simulink model "Steuerung"  (R2018a)
settings: Solver=ode1  StartTime=0.0  StopTime=inf  FixedStep=1/10  RelTol=1e-3  EnableMultiTasking=on
undefined symbols (not defined in the file or in its folder): gray
libraries: simulink x3, visiontransforms x2, PiCar_library x1, visiontextngfix x1, visionanalysis x1, visionstatistics x1, embdlinuxlib x1, visionsinks x1
settings Model: SimulationMode=external  Creator=raspberry  LastModifiedBy=jonaseckhoff
settings SolverCC: PositivePriorityOrder=on
settings OptimizationCC: PassReuseOutputArgsAs=Individual arguments  MaxStackSize=64
settings DebuggingCC: ParameterTunabilityLossMsg=error
settings HardwareCC: ProdBitPerPointer=32  ProdBitPerSizeT=32  ProdBitPerPtrDiffT=32  ProdLargestAtomicInteger=Long  ProdLargestAtomicFloat=Double  ProdWordSize=32  ProdHWDeviceType=ARM Compatible->ARM Cortex
settings SFSimCC: MATLABDynamicMemAlloc=off
settings RTWCC: SystemTargetFile=ert.tlc  HardwareBoard=Raspberry Pi  TLCOptions="-aInlineSetEventsForThisBaseRateFcn=TLC_FALSE -aSuppressMultiTaskScheduler=TLC_FALSE  -aRateBasedStepFcn=0"  TemplateMakefile=ert_default_tmf  Toolchain=GNU GCC Raspberry Pi
settings RTWCC: CustomTerminator=|
  | /* Send ALL_LED_OFF Signal to all PWM driver chip address
  | See PCA9685 user manual, section 7.3.4
  | Set Chip in sleep mode, section 7.3.1
  | Reset the PWM ON/OFF states for all LEDs */
  | 
  | int fd;
  | 
  | fd = wiringPiI2CSetup(0x70);
  | wiringPiI2CWriteReg8(fd, 0x00, 0x11); // sleep mode
  | wiringPiI2CWriteReg8(fd, 0xFD, 0x10); // all LED off
  | wiringPiI2CWriteReg8(fd, 0xFC, 0x00);
  | wiringPiI2CWriteReg8(fd, 0xFB, 0x00);
  | wiringPiI2CWriteReg8(fd, 0xFA, 0x00);
settings CodeAppCC: ForceParamTrailComments=on  IgnoreCustomStorageClasses=off  OperatorAnnotations=on  SimulinkDataObjDesc=on  SFDataObjDesc=on  MATLABFcnDesc=on  InsertBlockDesc=on  StateflowObjectComments=on  MATLABSourceComments=on
settings ERTTargetCC: SupportVariableSizeSignals=on

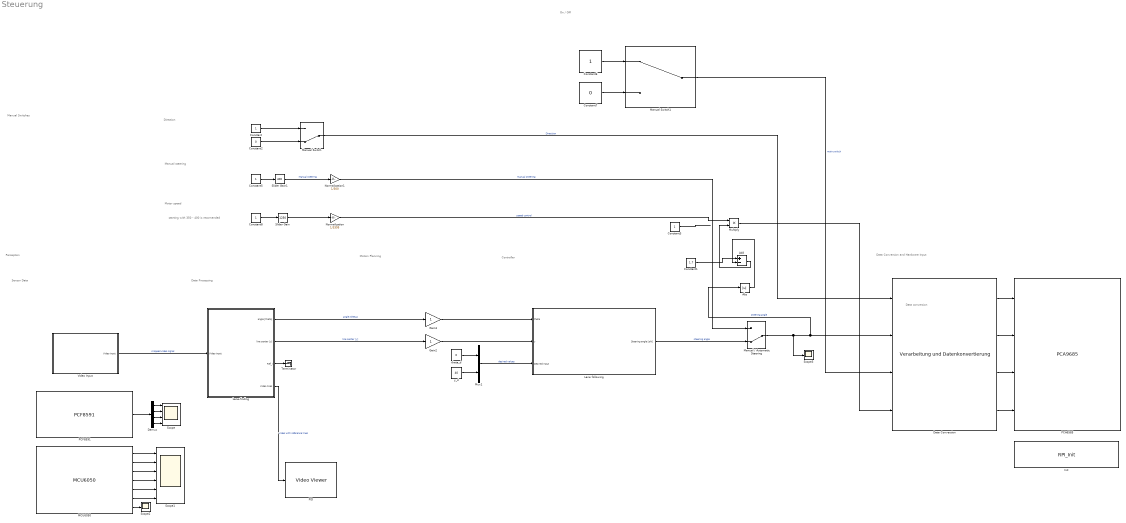
== system Steuerung ==
  note: starting with 350 - 400 is recomended
  note: Data Conversion and Hardware Input
  note: Data conversion
  note: Manual Switches
  note: Motion Planning
  note: Perception
  note: Controller
  note: Data Processing
  note: Sensor Data
  note: Manual steering
  note: Motor speed
  note: Direction
  note: On / Off
  Abs : Abs
  Add : Sum  Inputs=+-
  Constant{,3,5..6,8} (5 alike) : Constant
  Constant1 : Constant  Value=1.7
  Constant2 : Constant  Value=0
  Constant7 : Constant  Value=0
  Data Conversion : PiCar_library/Verarbeitung und Datenkonvertierung
      link override Gain1: Gain=340
  Demux : Demux
  Gain2 : Gain
  Gain3 : Gain
  Init : S-Function  Priority=1  InitFcn=try, set_param(gcb,'FunctionName','RPI_Init'), end  FunctionName=RPI_Init  SFunctionModules=RPI_Init_wrapper  SFunctionDeploymentMode=off  EnableBusSupport=off  mask(S-Function Builder){}
      mask help: Simulink:masks:SFunctionBuilder_MD
      mask init:
      | val = [[.9  0.75 0.75 1 1 .9 .9 1]',[1 1 0.75 0.75 .9 .9 1 .9]'];try , sys = get_param(gcb,'SfunBuilderFcnName');if isempty(sys), sys = get_param(gcb,'FunctionName'); end,catch, sys = get_param(gcb,'FunctionName'); end
      settings: CopyFcn=set_param(gcbh,'LinkStatus','none')  PreSaveFcn=try, set_param(gcb,'FunctionName','RPI_Init'), end  OpenFcn=sfunctionwizard(gcbh)
      mask Display:
      | plot(val(:,1),val(:,2))
      | disp(sys)
  Lane following : Subsystem  AncestorBlock=PiCar_library/Lane following
  Lane-finding : Subsystem  AncestorBlock=PiCar_library/Lane-finding
  MCU6050 : S-Function  InitFcn=try, set_param(gcb,'FunctionName','MCU6050'), end  FunctionName=MCU6050  SFunctionModules=MCU6050_wrapper  SFunctionDeploymentMode=off  EnableBusSupport=off  mask(S-Function Builder){}
      mask help: Simulink:masks:SFunctionBuilder_MD
      mask init: same as Steuerung/Init
      settings: CopyFcn=set_param(gcbh,'LinkStatus','none')  PreSaveFcn=try, set_param(gcb,'FunctionName','MCU6050'), end  OpenFcn=sfunctionwizard(gcbh)
      mask Display: plot(val(:,1),val(:,2)),disp(sys), port_label('output',1,'ax'), port_label('output',2,'ay'), port_label('output',3,'az'), port_label('output',4,'omx'), port_label('output',5,'omy'), port_label('output',6,'omz'), port_label('output',7,'temp')
  Manual / Automatic Steering : ManualSwitch  CurrentSetting=0
  Manual Switch : ManualSwitch  CurrentSetting=0
  Manual Switch1 : ManualSwitch
  Multiply : Product
  Mux1 : Mux  Inputs=2
  Normalization : Gain  Gain=1/3395
  Normalization1 : Gain  Gain=1/300
  PCA6585 : S-Function  InitFcn=try, set_param(gcb,'FunctionName','PCA9685'), end  FunctionName=PCA9685  SFunctionModules=PCA9685_wrapper  SFunctionDeploymentMode=off  EnableBusSupport=off  mask(S-Function Builder){}
      mask help: Simulink:masks:SFunctionBuilder_MD
      mask init: same as Steuerung/Init
      settings: CopyFcn=set_param(gcbh,'LinkStatus','none')  PreSaveFcn=try, set_param(gcb,'FunctionName','PCA9685'), end  OpenFcn=sfunctionwizard(gcbh)
      mask Display: plot(val(:,1),val(:,2)),disp(sys), port_label('input',1,'IN_1'), port_label('input',2,'IN_2'), port_label('input',3,'PWM'), port_label('input',4,'SERVO')
  PCF8591 : S-Function  InitFcn=try, set_param(gcb,'FunctionName','PCF8591'), end  FunctionName=PCF8591  SFunctionModules=PCF8591_wrapper  SFunctionDeploymentMode=off  EnableBusSupport=off  mask(S-Function Builder){}
      mask help: Simulink:masks:SFunctionBuilder_MD
      mask init: same as Steuerung/Init
      settings: CopyFcn=set_param(gcbh,'LinkStatus','none')  PreSaveFcn=try, set_param(gcb,'FunctionName','PCF8591'), end  OpenFcn=sfunctionwizard(gcbh)
      mask Display: plot(val(:,1),val(:,2)),disp(sys), port_label('output',1,'PCF8591_out')
  PID : VideoViewer  colormapValue=gray(256)  FigPos=[241 558 555 306]
  Scope : Scope  NumInputPorts=4
  Scope1 : Scope  NumInputPorts=6
  Scope2 : Scope
  Scope3 : Scope
  Slider Gain : simulink/Math Operations/Slider Gain  gain=1250  low=0  high=3395
  Slider Gain1 : simulink/Math Operations/Slider Gain  gain=400  low=-400  high=400
  Terminator : Terminator
  Video Input : Subsystem  AncestorBlock=PiCar_library/Video Input
  theta_d : Constant  Value=0
  y_d : Constant  Value=40
  wires:
  Constant/1 -> Manual Switch/1
  Constant2/1 -> Manual Switch/2
  Constant7/1 -> Manual Switch1/2
  Constant6/1 -> Manual Switch1/1
  Constant8/1 -> Slider Gain/1
  Slider Gain1/1 -> Normalization1/1  "Manual steering"
  Constant5/1 -> Slider Gain1/1
  Lane-finding/2(line center [y]) -> Gain2/1  "line center [y]"
  Demux/3 -> Scope/3
  Demux/4 -> Scope/4
  PCF8591/1 -> Demux/1
  MCU6050/2 -> Scope1/2
  MCU6050/3 -> Scope1/3
  MCU6050/1 -> Scope1/1
  MCU6050/4 -> Scope1/4
  MCU6050/5 -> Scope1/5
  MCU6050/6 -> Scope1/6
  MCU6050/7 -> Scope2/1
  Manual Switch/1 -> Data Conversion/1  "Direction"
  Manual / Automatic Steering/1 -> Abs/1, Data Conversion/2, Scope3/1  "steering angle"
  Manual Switch1/1 -> Data Conversion/3  "main switch"
  Data Conversion/1 -> PCA6585/1
  Data Conversion/2 -> PCA6585/2
  Data Conversion/3 -> PCA6585/3
  Data Conversion/4 -> PCA6585/4
  Lane-finding/1(angle [theta]) -> Gain3/1  "angle [theta]"
  Slider Gain/1 -> Normalization/1
  Lane-finding/3(Ref_I) -> Terminator/1
  Lane-finding/4(Video lines) -> PID/1  "video with reference lines"
  Normalization/1 -> Multiply/1  "speed control"
  y_d/1 -> Mux1/2
  theta_d/1 -> Mux1/1
  Mux1/1 -> Lane following/3(Desired input)  "desired values"
  Normalization1/1 -> Manual / Automatic Steering/1  "manual steering"
  Demux/1 -> Scope/1
  Demux/2 -> Scope/2
  Gain3/1 -> Lane following/1(theta)
  Gain2/1 -> Lane following/2(y)
  Lane following/1(Steering angle [phi]) -> Manual / Automatic Steering/2  "steering angle"
  Video Input/1(Video Input) -> Lane-finding/1(Video input)  "cropped video signal"
  Abs/1 -> Add/2
  Constant1/1 -> Add/1
  Multiply/1 -> Data Conversion/4
  Constant3/1 -> ?
  Add/1 -> Multiply/2

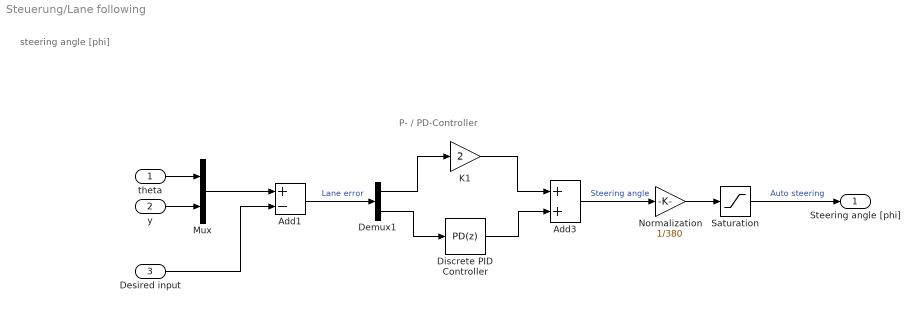
== system Steuerung/Lane following ==
  note: steering angle [phi]
  note: P- / PD-Controller
  theta : Inport
  y : Inport  Port=2
  Desired input : Inport  Port=3
  Add1 : Sum  Inputs=+-
  Add3 : Sum
  Demux1 : Demux  Outputs=2
  Discrete PID Controller : simulink/Continuous/PID Controller  Controller=PD  TimeDomain=Discrete-time  SampleTime=-1  IntegratorMethod=Forward Euler  FilterMethod=Forward Euler  Form=Parallel  UseFilter=off  ControllerParametersSource=internal  P=18  I=1.5  D=1.5  N=100  InitialConditionSource=internal  InitialConditionForIntegrator=0  InitialConditionForFilter=0  ExternalReset=none  LimitOutput=off  UpperSaturationLimit=inf  LowerSaturationLimit=-inf  LinearizeAsGain=off  AntiWindupMode=none  Kb=1  TrackingMode=off  Kt=1  PParamMin=[]  PParamMax=[]  IParamMin=[]  IParamMax=[]  DParamMin=[]  DParamMax=[]  NParamMin=[]  NParamMax=[]  KbParamMin=[]  KbParamMax=[]  KtParamMin=[]  KtParamMax=[]  POutMin=[]  POutMax=[]  IOutMin=[]  IOutMax=[]  DOutMin=[]  DOutMax=[]  NOutMin=[]  NOutMax=[]  KbOutMin=[]  KbOutMax=[]  KtOutMin=[]  KtOutMax=[]  IntegratorOutMin=[]  IntegratorOutMax=[]  FilterOutMin=[]  FilterOutMax=[]  SumOutMin=[]  SumOutMax=[]  SumI1OutMin=[]  SumI1OutMax=[]  SumI2OutMin=[]  SumI2OutMax=[]  SumI3OutMin=[]  SumI3OutMax=[]  SumDOutMin=[]  SumDOutMax=[]  SaturationOutMin=[]  SaturationOutMax=[]  IntegratorContinuousStateAttributes=''  IntegratorStateMustResolveToSignalObject=off  IntegratorRTWStateStorageClass=Auto  FilterContinuousStateAttributes=''  FilterStateMustResolveToSignalObject=off  FilterRTWStateStorageClass=Auto  DifferentiatorICPrevScaledInput=0  DifferentiatorOutMin=[]  DifferentiatorOutMax=[]  FilterDiffOutCoefMin=[]  FilterDiffOutCoefMax=[]  SumDenOutMin=[]  SumDenOutMax=[]  SumNumOutMin=[]  SumNumOutMax=[]  ReciprocalOutMin=[]  ReciprocalOutMax=[]  DivideOutMin=[]  DivideOutMax=[]  TunerSelectOption=Transfer Function Based (PID Tuner App)
  K1 : Gain  Gain=2
  Mux : Mux  Inputs=2
  Normalization : Gain  Gain=1/380
  Saturation : Saturate  UpperLimit=1  LowerLimit=-1
  Steering angle [phi] : Outport
  wires:
  theta/1 -> Mux/1
  y/1 -> Mux/2
  Mux/1 -> Add1/1
  Desired input/1 -> Add1/2
  Saturation/1 -> Steering angle [phi]/1  "Auto steering"
  Add3/1 -> Normalization/1  "Steering angle"
  Discrete PID Controller/1 -> Add3/2
  Demux1/2 -> Discrete PID Controller/1
  Add1/1 -> Demux1/1  "Lane error"
  Demux1/1 -> K1/1
  K1/1 -> Add3/1
  Normalization/1 -> Saturation/1

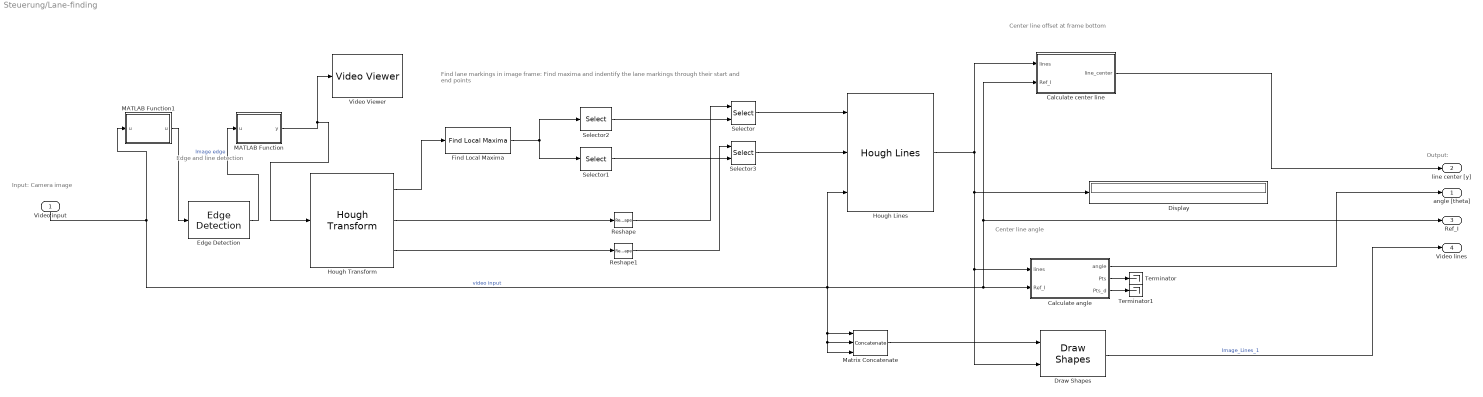
== system Steuerung/Lane-finding ==
  note: Output:
  note: Input: Camera image
  note: Edge and line detection
  note: Find lane markings in image frame:
      | Find maxima and indentify the lane markings through their start and end points
  note: Center line angle
  note: Center line offset at frame bottom
  Video input : Inport
  Calculate angle : MATLAB Function  TreatAsAtomicUnit=on
  Calculate center line : MATLAB Function  TreatAsAtomicUnit=on
  Display : Display
  Draw Shapes : visiontextngfix/Draw Shapes  shape=Lines  fill=off  lineWidth=1  fillClrSource=Specify via dialog  display=User-specified value  intensity=200  color=[0 0 255]  opacity=0.6  viewport=Entire image  antialiasing=off  inType=Obsolete  imagePorts=One multidimensional signal  prodOutputMode=Binary point scaling  prodOutputWordLength=32  prodOutputFracLength=14  memoryMode=Specify word length  memoryWordLength=16  memoryFracLength=14  roundingMode=Floor  overflowMode=off
      settings: SourceProductName=Computer Vision System Toolbox
  Edge Detection : visionanalysis/Edge Detection  method=Sobel  outputType=Binary image  userDefinedThreshold=off  thresholdSource=Input port  threshold=20  thresholdTuning=4  edgeThinning=off  threshold_canny=[0.25 0.60]  autoPercent=70  sigma=1  roundingMode=Floor  overflowMode=off  prodOutputMode=Binary point scaling  prodOutputWordLength=32  prodOutputFracLength=8  prodOutputSlope=2^-8  accumSlope=2^-8  outputSlope=2^-4
      settings: SourceProductName=Computer Vision System Toolbox  SourceProductBaseCode=VP
  Find Local Maxima : visionstatistics/Find Local Maxima  num_peaks=2  nhood_size=[5 7]  src_thresh=Obsolete9b  src_thresh_inuse=Specify via dialog  threshold=10  inputIsHough=off  dt_peak=uint32  isOutVarDim=on  dt_count=uint32
      settings: SourceProductName=Computer Vision System Toolbox  SourceProductBaseCode=VP
  Hough Lines : visiontransforms/Hough Lines  sineCompMethod=Trigonometric function  thetaRes=pi/180  firstCoeffMode=Specify word length  firstCoeffWordLength=16  firstCoeffFracLength=15  prodOutputMode=Binary point scaling  prodOutputWordLength=32  prodOutputFracLength=16  roundingMode=Nearest  overflowMode=on
      settings: SourceProductName=Computer Vision System Toolbox  SourceProductBaseCode=VP
  Hough Transform : visiontransforms/Hough Transform  theta_res=pi/180  rho_res=1  out_theta_rho=on  outdtmode=double  firstCoeffMode=Binary point scaling  firstCoeffWordLength=16  firstCoeffFracLength=14  secondCoeffMode=Binary point scaling  secondCoeffWordLength=32  secondCoeffFracLength=16  outputMode=Binary point scaling  outputWordLength=16  outputFracLength=0  accumMode=Binary point scaling  accumWordLength=32  accumFracLength=20  prodOutputMode=Binary point scaling  prodOutputWordLength=32  prodOutputFracLength=20  memoryMode=Binary point scaling  memoryWordLength=32  memoryFracLength=16  roundingMode=Nearest  overflowMode=on
      settings: SourceProductName=Computer Vision System Toolbox  SourceProductBaseCode=VP
  MATLAB Function : MATLAB Function  TreatAsAtomicUnit=on
  MATLAB Function1 : MATLAB Function  TreatAsAtomicUnit=on
  Matrix Concatenate : Concatenate  NumInputs=3  Mode=Multidimensional array  ConcatenateDimension=3
  Reshape : Reshape
  Reshape1 : Reshape
  Selector : Selector  IndexOptions=Index vector (port)  Indices=[1 3]  OutputSizes=1
  Selector1 : Selector  NumberOfDimensions=2  InputPortWidth=3  IndexOptions=Select all,Index vector (dialog)  Indices=[1 3],2  OutputSizes=1,1
  Selector2 : Selector  NumberOfDimensions=2  InputPortWidth=3  IndexOptions=Select all,Index vector (dialog)  Indices=[1 3],1  OutputSizes=1,1
  Selector3 : Selector  IndexOptions=Index vector (port)  Indices=[1 3]  OutputSizes=1
  Terminator : Terminator
  Terminator1 : Terminator
  Video Viewer : VideoViewer  FigPos=[312 917 418 304]
  angle [theta] : Outport
  line center [y] : Outport  Port=2
  Ref_I : Outport  Port=3
  Video lines : Outport  Port=4
  wires:
  Calculate center line/1(line_center) -> line center [y]/1
  Hough Lines/1 -> Calculate angle/1(lines), Draw Shapes/2, Display/1, Calculate center line/1(lines)
  Draw Shapes/1 -> Video lines/1  "Image_Lines_1"
  Calculate angle/1(angle) -> angle [theta]/1
  Matrix Concatenate/1 -> Draw Shapes/1
  Reshape1/1 -> Selector3/1
  Selector3/1 -> Hough Lines/2
  Reshape/1 -> Selector/1
  Selector/1 -> Hough Lines/1
  Find Local Maxima/1 -> Selector1/1, Selector2/1
  Selector2/1 -> Selector/2
  Selector1/1 -> Selector3/2
  Hough Transform/1 -> Find Local Maxima/1
  Hough Transform/3 -> Reshape1/1
  Hough Transform/2 -> Reshape/1
  Video input/1 -> MATLAB Function1/1("u "), Matrix Concatenate/3, Matrix Concatenate/2, Matrix Concatenate/1, Hough Lines/3, Ref_I/1, Calculate center line/2(Ref_I), Calculate angle/2(Ref_I)  "video input"
  Edge Detection/1 -> MATLAB Function/1(u)  "Image edge"
  Calculate angle/3(Pts_d) -> Terminator1/1
  Calculate angle/2(Pts) -> Terminator/1
  MATLAB Function/1(y) -> Video Viewer/1, Hough Transform/1
  MATLAB Function1/1(u) -> Edge Detection/1

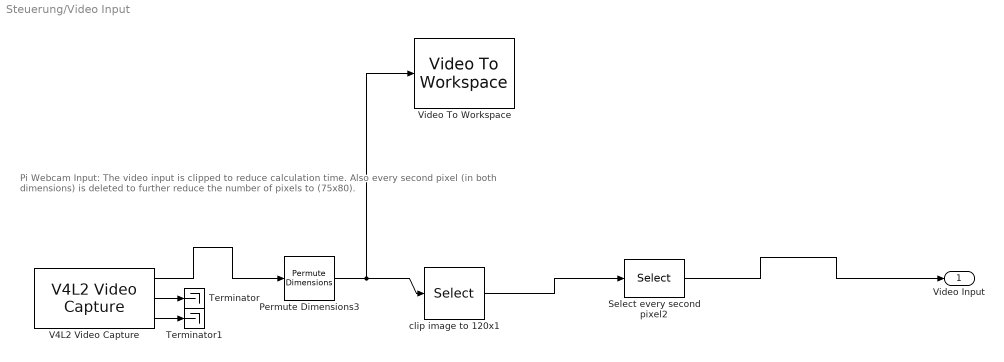
== system Steuerung/Video Input ==
  note: Pi Webcam Input:
      | The video input is clipped to reduce calculation time. Also every second pixel (in both dimensions) is deleted to further reduce the number of pixels
      | to (75x80).
  Permute Dimensions3 : PermuteDimensions
  Select every second pixel2 : Selector  NumberOfDimensions=2  InputPortWidth=3  IndexOptions=Select all,Index vector (dialog)  Indices=[1:2:80],[1:2:160]  OutputSizes=1,1
  Terminator : Terminator
  Terminator1 : Terminator
  V4L2 Video Capture : embdlinuxlib/V4L2 Video Capture  m_devName='/dev/video0'  roi=[0, 0, 640, 480]  imSizeSelection=320x240  imSize=[640, 480]  pixelFormat=YCbCr 4:2:2  pixelOrder=Planar  sampleTime=1/10  simOutput=Colorbars  blockPlatform=Raspberry Pi
      settings: SourceProductName=Simulink Support Package for Raspberry Pi Hardware  SourceProductBaseCode=RASPPI
  Video To Workspace : visionsinks/Video To Workspace  VariableName=vout  NumInputs=1  DataLimit=1000  DecimationFactor=1  LogFi=off  InPortLabels=R|G|B
      settings: SourceProductName=Computer Vision System Toolbox  SourceProductBaseCode=VP
  clip image to 120x1 : Selector  NumberOfDimensions=2  InputPortWidth=3  IndexOptions=Index vector (dialog),Index vector (dialog)  Indices=[166:1:216],[1:2:320]  OutputSizes=1,160
  Video Input : Outport
  wires:
  Select every second pixel2/1 -> Video Input/1
  V4L2 Video Capture/3 -> Terminator1/1
  V4L2 Video Capture/2 -> Terminator/1
  clip image to 120x1/1 -> Select every second pixel2/1
  Permute Dimensions3/1 -> Video To Workspace/1, clip image to 120x1/1
  V4L2 Video Capture/1 -> Permute Dimensions3/1

== matlab function Steuerung/Lane-finding/Calculate angle ==
  data: lines input; angle output; Pts output; Pts_d output; Ref_I input
function [angle, Pts, Pts_d] = angle(lines, Ref_I)

IMAGE_SIZE = size(Ref_I);
IMAGE_HEIGHT = IMAGE_SIZE(1);
IMAGE_WIDTH = IMAGE_SIZE(2);
points = zeros(2,4);

% Sorting the lines
if double(lines(1,1)) < double(lines(2,1))
    points(1,:) = lines(1,:);
    points(2,:) = lines(2,:);
else
    points(1,:) = lines(2,:);
    points(2,:) = lines(1,:);
end

% Calculate the lane center, top and bottom
x_center = double((points(1,:) + points(2,:))/2);

% Calculate the angle of the centerline: 0 -> vertical
angle = atan((x_center(3) - x_center(1))/IMAGE_HEIGHT);

% Auxilliary lines
Pts = int32([x_center(1), 1, x_center(3), 75]);
Pts_d = int32([IMAGE_WIDTH/2, 1, IMAGE_WIDTH/2, 75]);

% angles = atan2d(double((lines(:,1) - lines(:,3))), -double(lines(:,2) - lines(:,4)));

== matlab function Steuerung/Lane-finding/Calculate center line ==
  data: lines input; line_center output; Ref_I input
function line_center = center(lines, Ref_I)

IMAGE_SIZE = size(Ref_I);
IMAGE_HEIGHT = IMAGE_SIZE(1);
IMAGE_WIDTH = IMAGE_SIZE(2);
points = zeros(2,4);

% Sorting the lines
if double(lines(1,1)) < double(lines(2,1))
    points(1,:) = lines(1,:);
    points(2,:) = lines(2,:);
else
    points(1,:) = lines(2,:);
    points(2,:) = lines(1,:);
end

% Calculate the lane center, top and bottom
x_center = double((points(1,:) + points(2,:))/2);

% Output the lane center at the bottom of the picture
line_center = x_center(3);

== matlab function Steuerung/Lane-finding/MATLAB Function ==
  data: u input; y output
function y = fcn(u)
y=u;
for i=1:size(u,2)/2
    for j=1:floor(size(u,1))
        if i+j<floor(size(u,2)/2)
            y(j,i)=false;
            y(j,size(u,2)-i)=false;
        end
    end
end

end

== matlab function Steuerung/Lane-finding/MATLAB Function1 ==
  data: u input; u output
function u = fcn(u)

for i=1:size(u,1)
    for j=1:size(u,2)
        if (u(i,j))<150
            u(i,j)=uint8(0);
        end
    end
end


end
